simulink model "LIN_Edge"  (R2016b)
settings: Solver=FixedStepAuto  StartTime=0.0  StopTime=10  FixedStep=0.001  RelTol=1e-3
values from neighbouring files (symbols this model uses):
  A = [0, 1, 0; m*l_C*g*sqrt(2)/I_K, -C_psi/I_K, C_psi/I_K; 0, C_psi/I_R, -C_psi/I_R]    [ParameterInit.m]
  Ad = SSd.A    [ParameterInit.m]
  Ao = [SSd.A, zeros(3,3); zeros(3,3), eye(3)]    [controller_design_lqr.m]
  B = [0; -1/I_K; 1/I_R]    [ParameterInit.m]
  Bd = SSd.B    [ParameterInit.m]
  Bo = [SSd.B; zeros(3,1)]    [controller_design_lqr.m]
  C = [0, 1, 0; 0, 0, 1]    [ParameterInit.m]
  Cd = SSd.C    [ParameterInit.m]
  Co = [eye(3), eye(3)]    [controller_design_lqr.m]
  Kd = dlqr(SSd.A, SSd.B, Q, R)    [controller_design_lqr.m]
  Ld = (dlqr(SSd.A', SSd.C', Q, R))'    [controller_design_lqr.m]
  Lo = dlqr(Ao', Co', Q, R)'    [controller_design_lqr.m]
  Ta = 0.02    [ParameterInit.m]
  x_0 = [0.07; 0; 0]    [SimulinkInit.m]
  x_offset = [0.01; 0; 0]    [SimulinkInit.m]
libraries: simulink x1
settings Model: Creator=michael  LastModifiedBy=michael

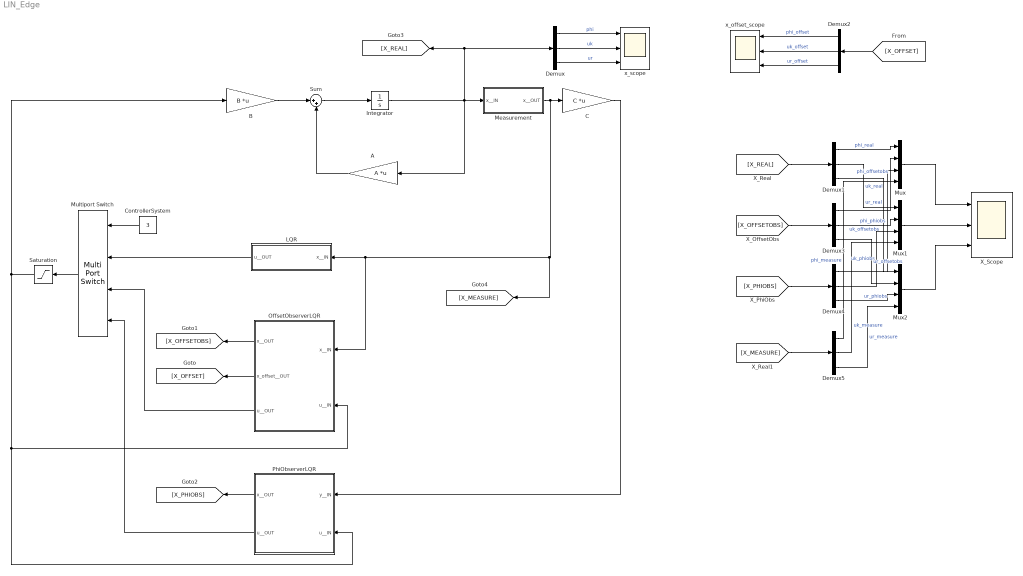
== system LIN_Edge ==
  A : Gain  Gain=A  Multiplication=Matrix(K*u) (u vector)
  B : Gain  Gain=B  Multiplication=Matrix(K*u) (u vector)
  C : Gain  Gain=C  Multiplication=Matrix(K*u) (u vector)
  ControllerSystem : Constant  Value=3
  Demux{,1..5} (6 alike) : Demux  Outputs=3
  Integrator : Integrator  InitialCondition=x_0
  LQR : Subsystem
  Measurement : Subsystem
  Multiport Switch : MultiPortSwitch
  Mux : Mux
  Mux1 : Mux
  Mux2 : Mux
  OffsetObserverLQR : Subsystem
  PhiObserverLQR : Subsystem
  Saturation : Saturate  UpperLimit=0.11  LowerLimit=-0.11
  Sum : Sum  Inputs=|++
  X_Scope : Scope  NumInputPorts=3
  x_offset_scope : Scope  NumInputPorts=3
  x_scope : Scope  NumInputPorts=3
  wires:
  B/1 -> Sum/1
  Sum/1 -> Integrator/1
  A/1 -> Sum/2
  Integrator/1 -> Demux/1, [X_REAL], Measurement/1(x__IN), A/1
  Demux/1 -> x_scope/1  "phi"
  Demux/2 -> x_scope/2  "uk"
  Demux/3 -> x_scope/3  "ur"
  Demux2/1 -> x_offset_scope/1  "phi_offset"
  Demux2/2 -> x_offset_scope/2  "uk_offset"
  Demux2/3 -> x_offset_scope/3  "ur_offset"
  Measurement/1(x__OUT) -> [X_MEASURE], OffsetObserverLQR/1(x__IN), LQR/1(x__IN), C/1
  Multiport Switch/1 -> Saturation/1
  LQR/1(u__OUT) -> Multiport Switch/2
  ControllerSystem/1 -> Multiport Switch/1
  [X_OFFSET] -> Demux2/1
  OffsetObserverLQR/2(x_offset__OUT) -> [X_OFFSET]
  OffsetObserverLQR/1(x__OUT) -> [X_OFFSETOBS]
  OffsetObserverLQR/3(u__OUT) -> Multiport Switch/3
  Saturation/1 -> B/1, OffsetObserverLQR/2(u__IN), PhiObserverLQR/2(u__IN)
  PhiObserverLQR/1(x__OUT) -> [X_PHIOBS]
  PhiObserverLQR/2(u__OUT) -> Multiport Switch/4
  [X_REAL] -> Demux1/1
  [X_OFFSETOBS] -> Demux3/1
  [X_PHIOBS] -> Demux4/1
  Demux1/1 -> Mux/1  "phi_real"
  Demux3/1 -> Mux/2  "phi_offsetobs"
  Demux4/1 -> Mux/3  "phi_phiobs"
  Demux1/2 -> Mux1/1  "uk_real"
  Demux3/2 -> Mux1/2  "uk_offsetobs"
  Demux4/2 -> Mux1/3  "uk_phiobs"
  Demux1/3 -> Mux2/1  "ur_real"
  Demux3/3 -> Mux2/2  "ur_offsetobs"
  Demux4/3 -> Mux2/3  "ur_phiobs"
  Mux1/1 -> X_Scope/2
  Mux/1 -> X_Scope/1
  Mux2/1 -> X_Scope/3
  C/1 -> PhiObserverLQR/1(y__IN)
  [X_MEASURE] -> Demux5/1
  Demux5/3 -> Mux2/4  "ur_measure"
  Demux5/2 -> Mux1/4  "uk_measure"
  Demux5/1 -> Mux/4  "phi_measure"

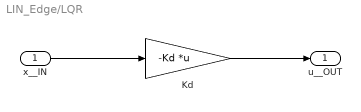
== system LIN_Edge/LQR ==
  x__IN : Inport  SampleTime=Ta
  Kd : Gain  Gain=-Kd  Multiplication=Matrix(K*u) (u vector)
  u__OUT : Outport
  wires:
  x__IN/1 -> Kd/1
  Kd/1 -> u__OUT/1

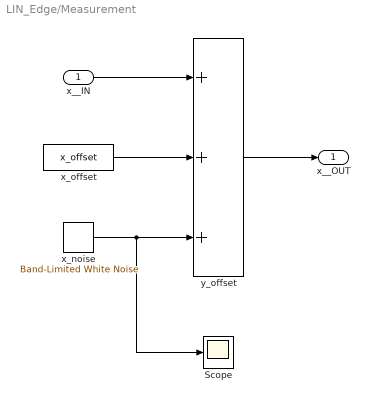
== system LIN_Edge/Measurement ==
  x__IN : Inport  SampleTime=Ta
  Scope : Scope
  x_noise : simulink/Sources/Band-Limited White Noise  Cov=y_noise  Ts=0.02  seed=[23341]
  x_offset : Constant  Value=x_offset
  y_offset : Sum  Inputs=+++
  x__OUT : Outport
  wires:
  x__IN/1 -> y_offset/1
  y_offset/1 -> x__OUT/1
  x_offset/1 -> y_offset/2
  x_noise/1 -> Scope/1, y_offset/3

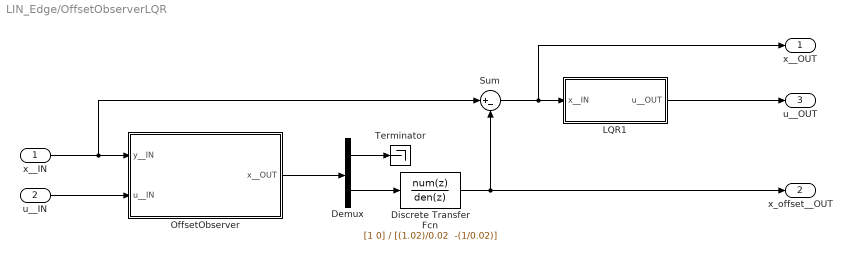
== system LIN_Edge/OffsetObserverLQR ==
  x__IN : Inport
  u__IN : Inport  Port=2
  Demux : Demux  Outputs=2
  Discrete Transfer Fcn : DiscreteTransferFcn  Numerator=[1 0]  Denominator="[(1.02)/0.02  -(1/0.02)]"
  LQR1 : Subsystem
  OffsetObserver : Subsystem
  Sum : Sum  Inputs=|+-
  Terminator : Terminator
  x__OUT : Outport
  x_offset__OUT : Outport  Port=2
  u__OUT : Outport  Port=3
  wires:
  x__IN/1 -> Sum/1, OffsetObserver/1(y__IN)
  u__IN/1 -> OffsetObserver/2(u__IN)
  OffsetObserver/1(x__OUT) -> Demux/1
  Demux/1 -> Terminator/1
  Sum/1 -> x__OUT/1, LQR1/1(x__IN)
  LQR1/1(u__OUT) -> u__OUT/1
  Demux/2 -> Discrete Transfer Fcn/1
  Discrete Transfer Fcn/1 -> x_offset__OUT/1, Sum/2

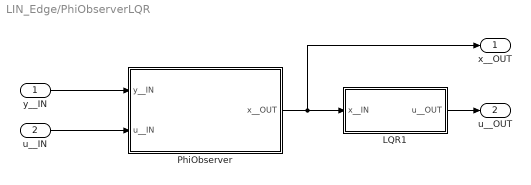
== system LIN_Edge/PhiObserverLQR ==
  y__IN : Inport
  u__IN : Inport  Port=2
  LQR1 : Subsystem
  PhiObserver : Subsystem
  x__OUT : Outport
  u__OUT : Outport  Port=2
  wires:
  LQR1/1(u__OUT) -> u__OUT/1
  PhiObserver/1(x__OUT) -> x__OUT/1, LQR1/1(x__IN)
  u__IN/1 -> PhiObserver/2(u__IN)
  y__IN/1 -> PhiObserver/1(y__IN)

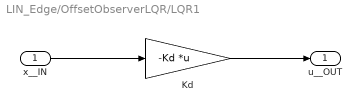
== system LIN_Edge/OffsetObserverLQR/LQR1 ==
  x__IN : Inport  SampleTime=Ta
  Kd : Gain  Gain=-Kd  Multiplication=Matrix(K*u) (u vector)
  u__OUT : Outport
  wires:
  Kd/1 -> u__OUT/1
  x__IN/1 -> Kd/1

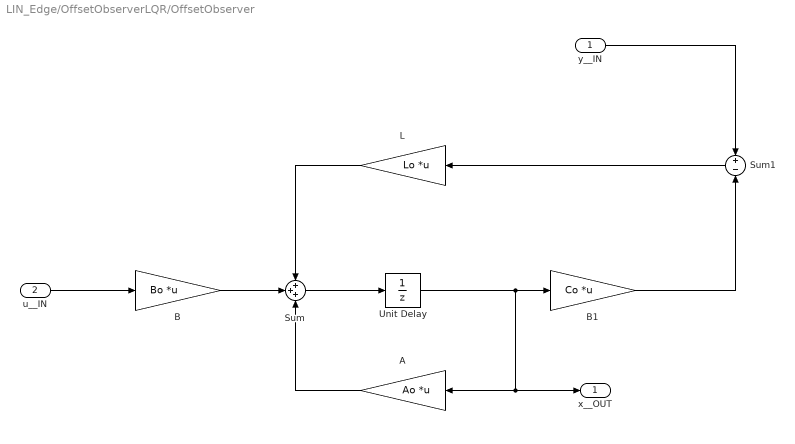
== system LIN_Edge/OffsetObserverLQR/OffsetObserver ==
  y__IN : Inport  SampleTime=Ta
  u__IN : Inport  Port=2  SampleTime=Ta
  A : Gain  Gain=Ao  Multiplication=Matrix(K*u) (u vector)
  B : Gain  Gain=Bo  Multiplication=Matrix(K*u) (u vector)
  B1 : Gain  Gain=Co  Multiplication=Matrix(K*u) (u vector)
  L : Gain  Gain=Lo  Multiplication=Matrix(K*u) (u vector)
  Sum : Sum  Inputs=+++
  Sum1 : Sum  Inputs=+|-
  Unit Delay : UnitDelay  InitialCondition=[x_0+x_offset; zeros(3,1)]  SampleTime=0.02
  x__OUT : Outport
  wires:
  u__IN/1 -> B/1
  B/1 -> Sum/2
  A/1 -> Sum/3
  L/1 -> Sum/1
  Sum/1 -> Unit Delay/1
  Unit Delay/1 -> B1/1, x__OUT/1, A/1
  Sum1/1 -> L/1
  B1/1 -> Sum1/2
  y__IN/1 -> Sum1/1

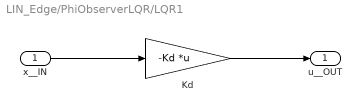
== system LIN_Edge/PhiObserverLQR/LQR1 ==
  x__IN : Inport  SampleTime=Ta
  Kd : Gain  Gain=-Kd  Multiplication=Matrix(K*u) (u vector)
  u__OUT : Outport
  wires:
  x__IN/1 -> Kd/1
  Kd/1 -> u__OUT/1

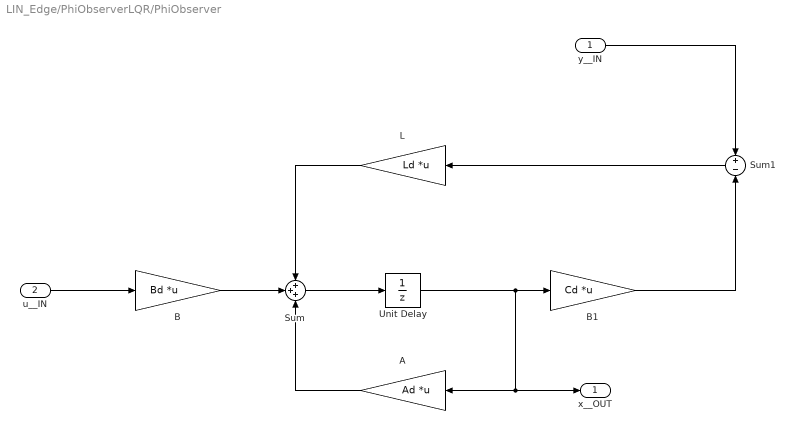
== system LIN_Edge/PhiObserverLQR/PhiObserver ==
  y__IN : Inport  SampleTime=Ta
  u__IN : Inport  Port=2  SampleTime=Ta
  A : Gain  Gain=Ad  Multiplication=Matrix(K*u) (u vector)
  B : Gain  Gain=Bd  Multiplication=Matrix(K*u) (u vector)
  B1 : Gain  Gain=Cd  Multiplication=Matrix(K*u) (u vector)
  L : Gain  Gain=Ld  Multiplication=Matrix(K*u) (u vector)
  Sum : Sum  Inputs=+++
  Sum1 : Sum  Inputs=+|-
  Unit Delay : UnitDelay  InitialCondition=[x_0+x_offset]  SampleTime=0.02
  x__OUT : Outport
  wires:
  y__IN/1 -> Sum1/1
  B1/1 -> Sum1/2
  Sum1/1 -> L/1
  Unit Delay/1 -> A/1, x__OUT/1, B1/1
  Sum/1 -> Unit Delay/1
  L/1 -> Sum/1
  A/1 -> Sum/3
  B/1 -> Sum/2
  u__IN/1 -> B/1
